simulink model "SIMULINKB"  (R2023b)
settings: Solver=VariableStepAuto  StartTime=0.0  StopTime=5000  FixedStep=0.001  RelTol=1e-3
values from neighbouring files (symbols this model uses):
  u0 = u_vec(i)    [Bodes.m]    (also in TP1.m = Qi/(a_salida*sqrt(2*g*h0)))
  x_e = [h0; 0]    [Bodes.m]    (also in TP1.m = 0.45)
libraries: cstblocks x1
settings Model: Creator=aghersin  LastModifiedBy=tomig
settings SolverCC: AlgebraicLoopSolver=TrustRegion
settings DataIOCC: ReturnWorkspaceOutputs=off
settings OptimizationCC: LifeSpan=inf
settings DebuggingCC: UnconnectedInputMsg=warning  UnconnectedOutputMsg=warning  UnconnectedLineMsg=warning  SFExecutionAtInitializationDiag=none  ArithmeticOperatorsInVariantConditions=warning
settings ModelReferenceCC: EnableRefExpFcnMdlSchedulingChecks=on
settings SFSimCC: SimUseLocalCustomCode=off  CustomCodeUndefinedFunction=UseInterfaceOnly
settings RTWCC: RTWUseLocalCustomCode=off  DLArmComputeVersion=19.05
settings CodeAppCC: StateflowObjectComments=on

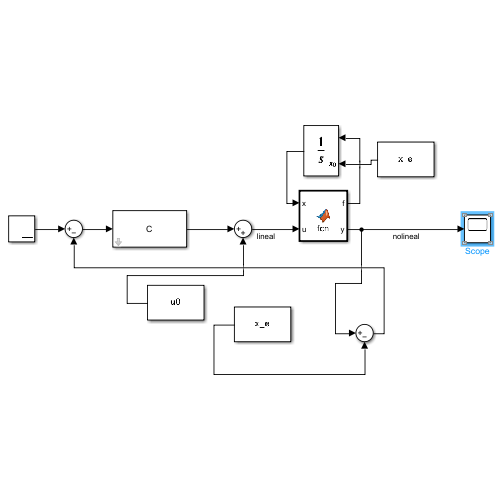
[thumbnail: Simulink's stored preview of the top-level diagram]
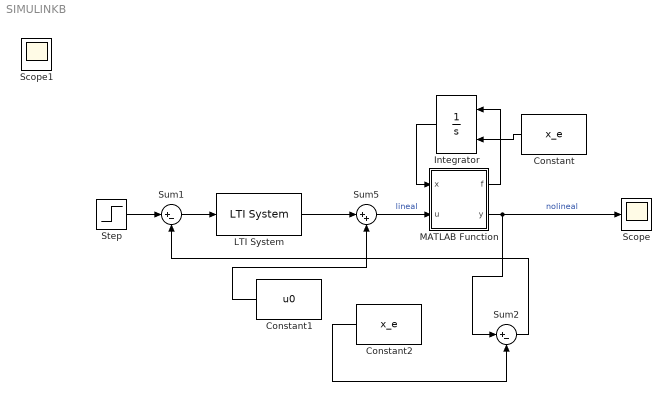
== system SIMULINKB ==
  Constant : Constant  Value=x_e
  Constant1 : Constant  Value=u0
  Constant2 : Constant  Value=x_e
  Integrator : Integrator  InitialConditionSource=external
  LTI System : cstblocks/LTI System  sys=C  IC=[]  PadeOrder=0
  MATLAB Function : MATLAB Function  TreatAsAtomicUnit=on
  Scope : Scope
  Step : Step  Before=0.45  After=0.35  SampleTime=0
  Sum1 : Sum  Inputs=|+-
  Sum2 : Sum  Inputs=|+-
  Sum5 : Sum  Inputs=|++
  Scope1 : Scope
  wires:
  Integrator/1 -> MATLAB Function/1(x)
  MATLAB Function/1(f) -> Integrator/1
  Constant/1 -> Integrator/2
  MATLAB Function/2(y) -> Scope/1, Sum2/1  "nolineal"
  Step/1 -> Sum1/1
  Sum1/1 -> LTI System/1
  LTI System/1 -> Sum5/1
  Sum5/1 -> MATLAB Function/2(u)  "lineal"
  Constant1/1 -> Sum5/2
  Constant2/1 -> Sum2/2
  Sum2/1 -> Sum1/2

== matlab function SIMULINKB/MATLAB Function ==
  data: x input; u input; f output; y output
function [f, y] = fcn(x, u)
    % Definición de constantes
    Qi = 8 * 0.001 / 60;  % Caudal constante de entrada (m^3/s)
    diam = 10.65 * 0.001; % Diámetro de la cañería de salida (m)
    l_chico = 0.1;        % Lado pequeño del tanque (m)
    l_grande = 0.4;       % Lado grande del tanque (m)
    h_tanque = 0.9;       % Altura del tanque (m)
    a_salida = pi * (diam / 2)^2; % Área de salida (m^2)
    g = 9.81;             % Gravedad (m/s^2)

    % Ecuación del sistema
    f = (Qi - (u * a_salida * sqrt(2 * g * x))) / ...
        ((l_chico)^2 + ((2 * l_chico * (l_grande - l_chico) * x) / h_tanque) + ...
        (((l_grande - l_chico) / h_tanque) * x)^2);
    
    % Salida del sistema
    y = x;
end
